simulink model "aerodinamica"  (Simulink 8.6)
settings: Solver=FixedStepAuto  StartTime=0  StopTime=150  FixedStep=1/5  RelTol=1e-3
model workspace: external: MATLAB Code (data not in the file)
values from neighbouring files (symbols this model uses):
  CD_alpha = 0.3840    (= 0.384)    [t37_data.m]
  CD_beta = [-1.5700	1.2300 ... (first row only)    [t37_data.m]
  CD_de = 0.0750    (= 0.075)    [t37_data.m]
  CD_flap = 0.0750    (= 0.075)    [t37_data.m]
  CD_ground_effect = [0.0000	0.8100 ... (first row only)    [t37_data.m]
  CD_mach = [0.0000	0.0000 ... (first row only)    [t37_data.m]
  CD_zero = [  -1.5700	1.5000 ... (first row only)    [t37_data.m]
  Cl_ail = [0.0000	0.1810 ... (first row only)    [t37_data.m]
  CL_alpha = [-0.2000	-0.6400 ... (first row only)    [t37_data.m]
  CL_alpha_dot = 2.0    (= 2)    [t37_data.m]
  Cl_beta = -0.0944    [t37_data.m]
  CL_elev = 0.5    [t37_data.m]
  CL_flap = 0.3500    (= 0.35)    [t37_data.m]
  CL_ground_effect = [0.0000	1.0610 ... (first row only)    [t37_data.m]
  Cl_p = -0.4420    (= -0.442)    [t37_data.m]
  CL_q = 4.1    [t37_data.m]
  Cl_r = 0.0926    [t37_data.m]
  Cl_rudder = 0.0150    (= 0.015)    [t37_data.m]
  Cm_alpha = -0.7000    (= -0.7)    [t37_data.m]
  Cm_alpha_dot = -6.9500    (= -6.95)    [t37_data.m]
  Cm_elev = [0.0000	-1.1200 ... (first row only)    [t37_data.m]
  Cm_q = -50.0000    (= -50)    [t37_data.m]
  Cm_zero = 0.0250    (= 0.025)    [t37_data.m]
  Cn_beta = 0.1106    [t37_data.m]
  Cn_p = -0.0243    [t37_data.m]
  Cn_r = -0.1390    (= -0.139)    [t37_data.m]
  Cn_rudder = -0.0365    [t37_data.m]
  Cnda = -0.0254    [t37_data.m]
  CY_beta = -0.3460    (= -0.346)    [t37_data.m]
  CY_p = -0.0827    [t37_data.m]
  CY_r = 0.3000    (= 0.3)    [t37_data.m]
  CY_rudder = 0.200    (= 0.2)    [t37_data.m]
  Sw = 182*0.09290304    (= 16.90835328)    [t37_data.m]
undefined symbols (not defined in the file): Bw, Cw
settings Model: Creator=willi  LastModifiedBy=willi
settings DataIOCC: SaveFormat=Dataset  SignalLoggingSaveFormat=Dataset
settings OptimizationCC: ExpressionDepthLimit=128
settings DebuggingCC: UnderspecifiedInitializationDetection=Simplified  MergeDetectMultiDrivingBlocksExec=error  SolverPrmCheckMsg=none  FcnCallInpInsideContextMsg=EnableAllAsError  StateNameClashWarn=none
settings HardwareCC: ProdBitPerPointer=64  ProdLargestAtomicFloat=Float  ProdIntDivRoundTo=Zero  ProdEndianess=LittleEndian  ProdWordSize=64  ProdHWDeviceType=Intel->x86-64 (Windows64)
settings GRTTargetCC: GeneratePreprocessorConditionals=Use local settings  CombineOutputUpdateFcns=on  GRTInterface=off

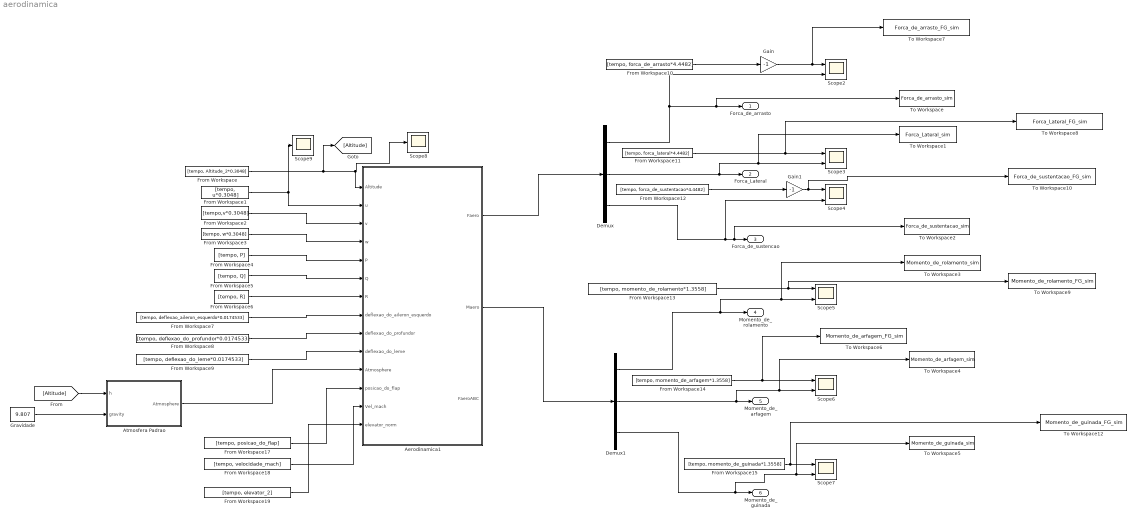
== system aerodinamica ==
  Aerodinamica1 : Subsystem  mask{flap=0, bw=Bw, cw=Cw, Sw=Sw}
      mask prompts: flap "Comando Flap (0, 1, 2 ou 3)"; bw "Comprimento da asa  - wingspan (m)"; cw "Corda media da asa (m)"; Sw "Area da asa (m2)"
  Atmosfera Padrao : Subsystem
  Demux : Demux  Outputs=3
  Demux1 : Demux  Outputs=3
  From Workspace : FromWorkspace  VariableName=[tempo, Altitude_2*0.3048]  SampleTime=0
  From Workspace1 : FromWorkspace  VariableName=[tempo, u*0.3048]  SampleTime=0
  From Workspace10 : FromWorkspace  VariableName=[tempo, forca_de_arrasto*4.4482]  SampleTime=0
  From Workspace11 : FromWorkspace  VariableName=[tempo, forca_lateral*4.4482]  SampleTime=0
  From Workspace12 : FromWorkspace  VariableName=[tempo, forca_de_sustentacao*4.4482]  SampleTime=0
  From Workspace13 : FromWorkspace  VariableName=[tempo, momento_de_rolamento*1.3558]  SampleTime=0
  From Workspace14 : FromWorkspace  VariableName=[tempo, momento_de_arfagem*1.3558]  SampleTime=0
  From Workspace15 : FromWorkspace  VariableName=[tempo, momento_de_guinada*1.3558]  SampleTime=0
  From Workspace17 : FromWorkspace  VariableName=[tempo, posicao_do_flap]  SampleTime=0
  From Workspace18 : FromWorkspace  VariableName=[tempo, velocidade_mach]  SampleTime=0
  From Workspace19 : FromWorkspace  VariableName=[tempo, elevator_2]  SampleTime=0
  From Workspace2 : FromWorkspace  VariableName=[tempo,v*0.3048]  SampleTime=0
  From Workspace3 : FromWorkspace  VariableName=[tempo, w*0.3048]  SampleTime=0
  From Workspace4 : FromWorkspace  VariableName=[tempo, P]  SampleTime=0
  From Workspace5 : FromWorkspace  VariableName=[tempo, Q]  SampleTime=0
  From Workspace6 : FromWorkspace  VariableName=[tempo, R]  SampleTime=0
  From Workspace7 : FromWorkspace  VariableName=[tempo, deflexao_aileron_esquerdo*0.0174533]  SampleTime=0
  From Workspace8 : FromWorkspace  VariableName=[tempo, deflexao_do_profundor*0.0174533]  SampleTime=0
  From Workspace9 : FromWorkspace  VariableName=[tempo, deflexao_do_leme*0.0174533]  SampleTime=0
  Gain : Gain  Gain=-1
  Gain1 : Gain  Gain=-1
  Gravidade : Constant  Value=9.807
  Scope{2..7} (6 alike) : Scope  NumInputPorts=2
  Scope8 : Scope
  Scope9 : Scope
  To Workspace : ToWorkspace  VariableName=Forca_de_arrasto_sim  SampleTime=-1
  To Workspace1 : ToWorkspace  VariableName=Forca_Lateral_sim  SampleTime=-1
  To Workspace10 : ToWorkspace  VariableName=Forca_de_sustentacao_FG_sim  SampleTime=-1
  To Workspace12 : ToWorkspace  VariableName=Momento_de_guinada_FG_sim  SampleTime=-1
  To Workspace2 : ToWorkspace  VariableName=Forca_de_sustentacao_sim  SampleTime=-1
  To Workspace3 : ToWorkspace  VariableName=Momento_de_rolamento_sim  SampleTime=-1
  To Workspace4 : ToWorkspace  VariableName=Momento_de_arfagem_sim  SampleTime=-1
  To Workspace5 : ToWorkspace  VariableName=Momento_de_guinada_sim  SampleTime=-1
  To Workspace6 : ToWorkspace  VariableName=Momento_de_arfagem_FG_sim  SampleTime=-1
  To Workspace7 : ToWorkspace  VariableName=Forca_de_arrasto_FG_sim  SampleTime=-1
  To Workspace8 : ToWorkspace  VariableName=Forca_Lateral_FG_sim  SampleTime=-1
  To Workspace9 : ToWorkspace  VariableName=Momento_de_rolamento_FG_sim  SampleTime=-1
  Forca_de_arrasto : Outport
  Forca_Lateral : Outport  Port=2
  Forca_de_sustencao : Outport  Port=3
  Momento_de_rolamento : Outport  Port=4
  Momento_de_arfagem : Outport  Port=5
  Momento_de_guinada : Outport  Port=6
  wires:
  From Workspace4/1 -> Aerodinamica1/5(P)
  From Workspace5/1 -> Aerodinamica1/6(Q)
  From Workspace6/1 -> Aerodinamica1/7(R)
  From Workspace7/1 -> Aerodinamica1/8("deflexao_do_aileron_esquerdo ")
  From Workspace8/1 -> Aerodinamica1/9("deflexao_do_profundor ")
  From Workspace9/1 -> Aerodinamica1/10(deflexao_do_leme)
  From Workspace1/1 -> Scope9/1, Aerodinamica1/2(u)
  From Workspace2/1 -> Aerodinamica1/3(v)
  From Workspace3/1 -> Aerodinamica1/4("w ")
  Gravidade/1 -> Atmosfera Padrao/2(gravity)
  Atmosfera Padrao/1(Atmosphere) -> Aerodinamica1/11(Atmosphere)
  [Altitude] -> Atmosfera Padrao/1(h)
  Aerodinamica1/1(Faero) -> Demux/1
  Demux/1 -> Scope2/2, To Workspace/1, Forca_de_arrasto/1
  Demux/2 -> To Workspace1/1, Scope3/2, Forca_Lateral/1
  Aerodinamica1/2(Maero) -> Demux1/1
  Demux/3 -> Scope4/2, To Workspace2/1, Forca_de_sustencao/1
  Demux1/2 -> Scope6/2, To Workspace4/1, Momento_de_arfagem/1
  Demux1/3 -> To Workspace5/1, Scope7/2, Momento_de_guinada/1
  Demux1/1 -> To Workspace3/1, Scope5/2, Momento_de_rolamento/1
  From Workspace14/1 -> Scope6/1, To Workspace6/1
  From Workspace15/1 -> To Workspace12/1, Scope7/1
  Gain/1 -> To Workspace7/1, Scope2/1
  From Workspace10/1 -> Gain/1
  Gain1/1 -> To Workspace10/1, Scope4/1
  From Workspace12/1 -> Gain1/1
  From Workspace11/1 -> To Workspace8/1, Scope3/1
  From Workspace17/1 -> Aerodinamica1/12(posicao_do_flap)
  From Workspace18/1 -> Aerodinamica1/13(Vel_mach)
  From Workspace13/1 -> To Workspace9/1, Scope5/1
  From Workspace/1 -> [Altitude], Scope8/1, Aerodinamica1/1(Altitude)
  From Workspace19/1 -> Aerodinamica1/14("elevator_norm ")

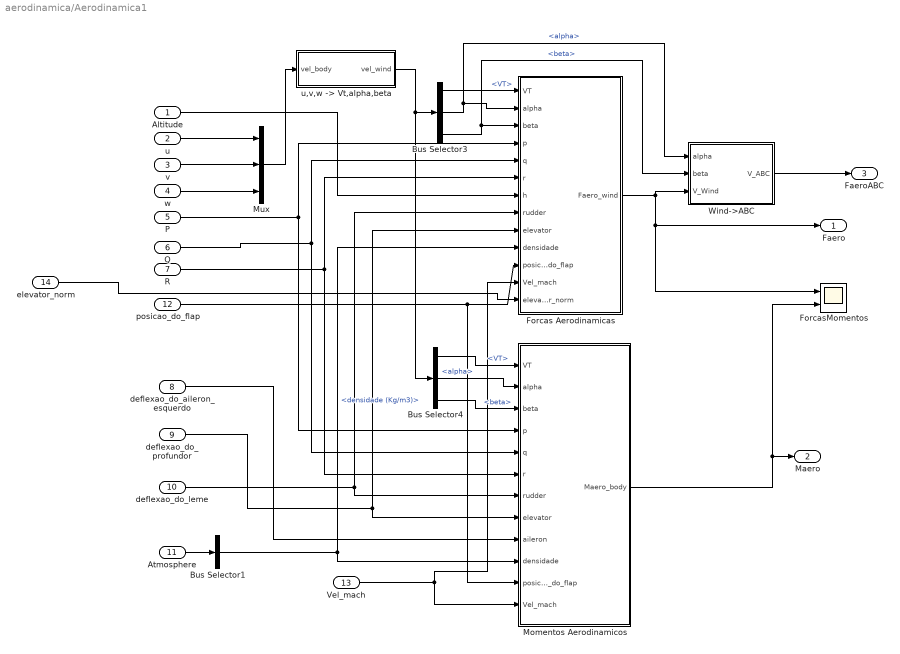
== system aerodinamica/Aerodinamica1 ==
  Altitude : Inport
  u : Inport  Port=2
  v : Inport  Port=3
  "w " : Inport  Port=4
  P : Inport  Port=5
  Q : Inport  Port=6
  R : Inport  Port=7
  "deflexao_do_aileron_esquerdo " : Inport  Port=8
  "deflexao_do_profundor " : Inport  Port=9
  deflexao_do_leme : Inport  Port=10
  Atmosphere : Inport  Port=11
  posicao_do_flap : Inport  Port=12
  Vel_mach : Inport  Port=13
  "elevator_norm " : Inport  Port=14
  Bus Selector1 : BusSelector  OutputSignals=densidade (Kg/m3)
  Bus Selector3 : BusSelector  OutputSignals=VT,alpha,beta
  Bus Selector4 : BusSelector  OutputSignals=VT,alpha,beta
  Forcas Aerodinamicas : Subsystem
  ForcasMomentos : Scope  NumInputPorts=2
  Momentos Aerodinamicos : Subsystem
  Mux : Mux  Inputs=3
  Wind->ABC : Subsystem
  "u,v,w -> Vt,alpha,beta" : Subsystem
  Faero : Outport
  Maero : Outport  Port=2
  FaeroABC : Outport  Port=3
  wires:
  Bus Selector1/1 -> Forcas Aerodinamicas/10(densidade), Momentos Aerodinamicos/10(densidade)  "<densidade (Kg/m3)>"
  Altitude/1 -> Forcas Aerodinamicas/7(h)
  P/1 -> Forcas Aerodinamicas/4(p), Momentos Aerodinamicos/4(p)
  Q/1 -> Forcas Aerodinamicas/5(q), Momentos Aerodinamicos/5(q)
  R/1 -> Forcas Aerodinamicas/6(r), Momentos Aerodinamicos/6(r)
  "deflexao_do_aileron_esquerdo "/1 -> Momentos Aerodinamicos/9(aileron)
  "deflexao_do_profundor "/1 -> Forcas Aerodinamicas/9(elevator), Momentos Aerodinamicos/8(elevator)
  deflexao_do_leme/1 -> Forcas Aerodinamicas/8(rudder), Momentos Aerodinamicos/7(rudder)
  Bus Selector3/1 -> Forcas Aerodinamicas/1(VT)  "<VT>"
  Bus Selector3/2 -> Forcas Aerodinamicas/2(alpha), Wind->ABC/1(alpha)  "<alpha>"
  Bus Selector3/3 -> Forcas Aerodinamicas/3(beta), Wind->ABC/2(beta)  "<beta>"
  Bus Selector4/1 -> Momentos Aerodinamicos/1(VT)  "<VT>"
  Bus Selector4/2 -> Momentos Aerodinamicos/2(alpha)  "<alpha>"
  Bus Selector4/3 -> Momentos Aerodinamicos/3(beta)  "<beta>"
  "u,v,w -> Vt,alpha,beta"/1(vel_wind) -> Bus Selector3/1, Bus Selector4/1
  u/1 -> Mux/1
  v/1 -> Mux/2
  "w "/1 -> Mux/3
  Mux/1 -> "u,v,w -> Vt,alpha,beta"/1(vel_body)
  Forcas Aerodinamicas/1(Faero_wind) -> Wind->ABC/3(V_Wind), ForcasMomentos/1, Faero/1
  Momentos Aerodinamicos/1(Maero_body) -> Maero/1, ForcasMomentos/2
  Atmosphere/1 -> Bus Selector1/1
  posicao_do_flap/1 -> Momentos Aerodinamicos/11(posicao_do_flap), Forcas Aerodinamicas/11("posicao_do_flap ")
  Vel_mach/1 -> Forcas Aerodinamicas/12(Vel_mach), Momentos Aerodinamicos/12(Vel_mach)
  "elevator_norm "/1 -> Forcas Aerodinamicas/13(elevator_norm)
  Wind->ABC/1(V_ABC) -> FaeroABC/1

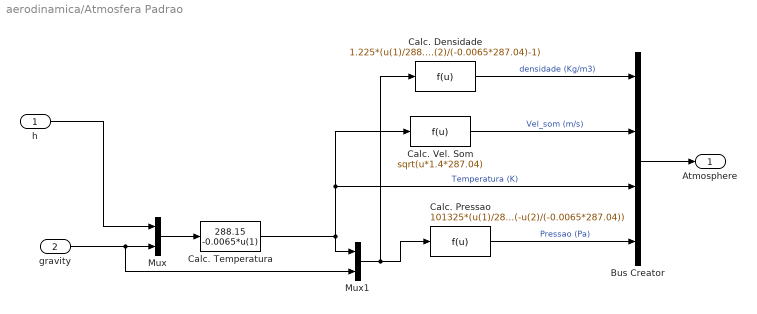
== system aerodinamica/Atmosfera Padrao ==
  h : Inport
  gravity : Inport  Port=2
  Bus Creator : BusCreator  Inputs=4
  Calc. Densidade : Fcn  Expr=1.225*(u(1)/288.15)^(-u(2)/(-0.0065*287.04)-1)
  Calc. Pressao : Fcn  Expr=101325*(u(1)/288.15)^(-u(2)/(-0.0065*287.04))
  Calc. Temperatura : Fcn  Expr=288.15 -0.0065*u(1)
  Calc. Vel. Som : Fcn  Expr=sqrt(u*1.4*287.04)
  Mux : Mux  Inputs=2
  Mux1 : Mux  Inputs=2
  Atmosphere : Outport
  wires:
  h/1 -> Mux/1
  gravity/1 -> Mux/2, Mux1/2
  Mux/1 -> Calc. Temperatura/1
  Mux1/1 -> Calc. Pressao/1, Calc. Densidade/1
  Calc. Temperatura/1 -> Mux1/1, Calc. Vel. Som/1, Bus Creator/3  "Temperatura (K)"
  Calc. Pressao/1 -> Bus Creator/4  "Pressao (Pa)"
  Calc. Densidade/1 -> Bus Creator/1  "densidade (Kg/m3)"
  Calc. Vel. Som/1 -> Bus Creator/2  "Vel_som (m/s)"
  Bus Creator/1 -> Atmosphere/1

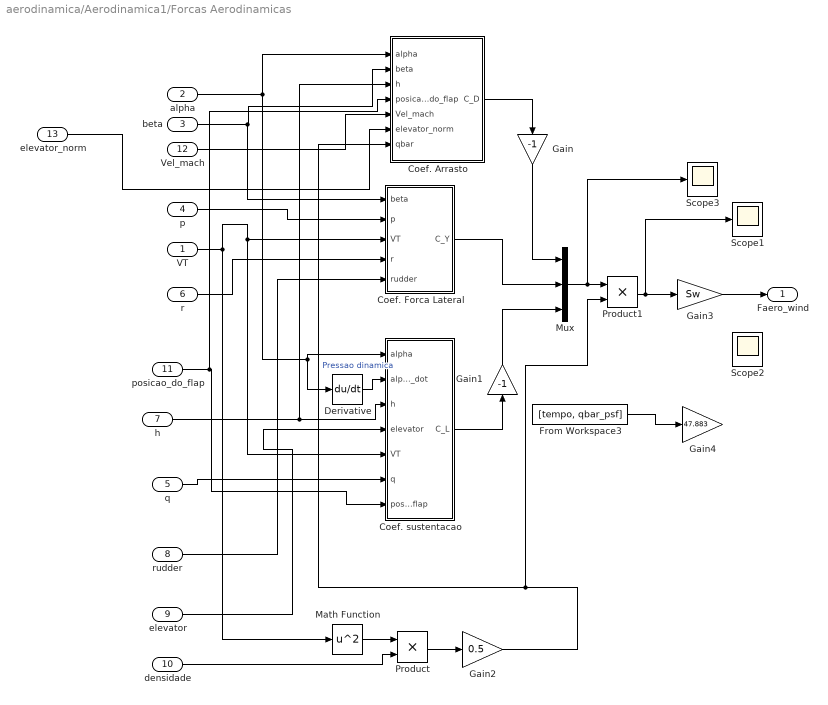
== system aerodinamica/Aerodinamica1/Forcas Aerodinamicas ==
  VT : Inport
  alpha : Inport  Port=2
  beta : Inport  Port=3
  p : Inport  Port=4
  q : Inport  Port=5
  r : Inport  Port=6
  h : Inport  Port=7
  rudder : Inport  Port=8
  elevator : Inport  Port=9
  densidade : Inport  Port=10
  "posicao_do_flap " : Inport  Port=11
  Vel_mach : Inport  Port=12
  elevator_norm : Inport  Port=13
  Coef. Arrasto : Subsystem
  Coef. Forca Lateral : Subsystem
  Coef. sustentacao : Subsystem
  Derivative : Derivative
  From Workspace3 : FromWorkspace  VariableName=[tempo, qbar_psf]  SampleTime=0
  Gain : Gain  Gain=-1  SaturateOnIntegerOverflow=on  OutDataTypeStr=Inherit: Same as input  ParamDataTypeStr=Inherit: Same as input
  Gain1 : Gain  Gain=-1  SaturateOnIntegerOverflow=on  OutDataTypeStr=Inherit: Same as input  ParamDataTypeStr=Inherit: Same as input
  Gain2 : Gain  Gain=0.5  SaturateOnIntegerOverflow=on  OutDataTypeStr=Inherit: Same as input  ParamDataTypeStr=Inherit: Same as input
  Gain3 : Gain  Gain=Sw  SaturateOnIntegerOverflow=on  OutDataTypeStr=Inherit: Same as input  ParamDataTypeStr=Inherit: Same as input
  Gain4 : Gain  Gain=47.883  SaturateOnIntegerOverflow=on  OutDataTypeStr=Inherit: Same as input  ParamDataTypeStr=Inherit: Same as input
  Math Function : Math  Operator=square  SaturateOnIntegerOverflow=on
  Mux : Mux  Inputs=3
  Product : Product  SaturateOnIntegerOverflow=on  OutDataTypeStr=Inherit: Same as first input
  Product1 : Product  SaturateOnIntegerOverflow=on  OutDataTypeStr=Inherit: Same as first input
  Scope1 : Scope
  Scope2 : Scope
  Scope3 : Scope
  Faero_wind : Outport
  wires:
  Coef. Arrasto/1(C_D) -> Gain/1
  Coef. Forca Lateral/1(C_Y) -> Mux/2
  alpha/1 -> Coef. Arrasto/1(alpha), Coef. sustentacao/1(alpha), Derivative/1
  beta/1 -> Coef. Arrasto/2(beta), Coef. Forca Lateral/1(beta)
  VT/1 -> Coef. Forca Lateral/3(VT), Coef. sustentacao/5(VT), Math Function/1
  p/1 -> Coef. Forca Lateral/2(p)
  q/1 -> Coef. sustentacao/6(q)
  r/1 -> Coef. Forca Lateral/4(r)
  h/1 -> Coef. Arrasto/3(h), Coef. sustentacao/3(h)
  rudder/1 -> Coef. Forca Lateral/5(rudder)
  elevator/1 -> Coef. sustentacao/4(elevator)
  Derivative/1 -> Coef. sustentacao/2(alpha_dot)
  Coef. sustentacao/1(C_L) -> Gain1/1
  Gain/1 -> Mux/1
  Gain1/1 -> Mux/3
  densidade/1 -> Product/2
  Math Function/1 -> Product/1
  Product/1 -> Gain2/1
  Mux/1 -> Scope3/1, Product1/1
  Product1/1 -> Scope1/1, Gain3/1
  Gain2/1 -> Product1/2, Coef. Arrasto/7(qbar)  "Pressao dinamica"
  Gain3/1 -> Faero_wind/1
  "posicao_do_flap "/1 -> Coef. Arrasto/4(posicao_do_flap), Coef. sustentacao/7("posicao_do_flap ")
  Vel_mach/1 -> Coef. Arrasto/5(Vel_mach)
  elevator_norm/1 -> Coef. Arrasto/6(elevator_norm)
  From Workspace3/1 -> Gain4/1

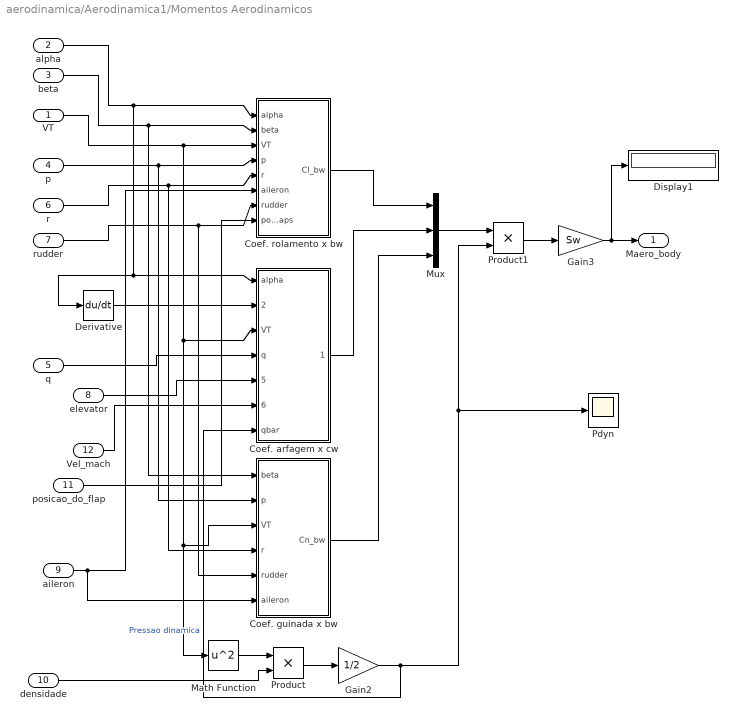
== system aerodinamica/Aerodinamica1/Momentos Aerodinamicos ==
  VT : Inport
  alpha : Inport  Port=2
  beta : Inport  Port=3
  p : Inport  Port=4
  q : Inport  Port=5
  r : Inport  Port=6
  rudder : Inport  Port=7
  elevator : Inport  Port=8
  aileron : Inport  Port=9
  densidade : Inport  Port=10
  posicao_do_flap : Inport  Port=11
  Vel_mach : Inport  Port=12
  Coef. arfagem x cw : Subsystem
  Coef. guinada x bw : Subsystem
  Coef. rolamento x bw : Subsystem
  Derivative : Derivative
  Display1 : Display
  Gain2 : Gain  Gain=1/2  SaturateOnIntegerOverflow=on  OutDataTypeStr=Inherit: Same as input  ParamDataTypeStr=Inherit: Same as input
  Gain3 : Gain  Gain=Sw  SaturateOnIntegerOverflow=on  OutDataTypeStr=Inherit: Same as input  ParamDataTypeStr=Inherit: Same as input
  Math Function : Math  Operator=square  SaturateOnIntegerOverflow=on
  Mux : Mux  Inputs=3
  Pdyn : Scope
  Product : Product  SaturateOnIntegerOverflow=on  OutDataTypeStr=Inherit: Same as first input
  Product1 : Product  SaturateOnIntegerOverflow=on  OutDataTypeStr=Inherit: Same as first input
  Maero_body : Outport
  wires:
  alpha/1 -> Coef. rolamento x bw/1(alpha), Coef. arfagem x cw/1(alpha), Derivative/1
  beta/1 -> Coef. rolamento x bw/2(beta), Coef. guinada x bw/1(beta)
  VT/1 -> Coef. rolamento x bw/3(VT), Coef. arfagem x cw/3(VT), Coef. guinada x bw/3(VT), Math Function/1
  p/1 -> Coef. rolamento x bw/4(p), Coef. guinada x bw/2(p)
  r/1 -> Coef. rolamento x bw/5(r), Coef. guinada x bw/4(r)
  Derivative/1 -> Coef. arfagem x cw/2(alpha_dot)
  q/1 -> Coef. arfagem x cw/4(q)
  rudder/1 -> Coef. rolamento x bw/7(rudder), Coef. guinada x bw/5(rudder)
  elevator/1 -> Coef. arfagem x cw/5(elevator)
  aileron/1 -> Coef. guinada x bw/6("aileron "), Coef. rolamento x bw/6(aileron)
  Mux/1 -> Product1/1
  Product1/1 -> Gain3/1
  Coef. rolamento x bw/1(Cl_bw) -> Mux/1
  Coef. arfagem x cw/1(Cm_cw) -> Mux/2
  Coef. guinada x bw/1(Cn_bw) -> Mux/3
  densidade/1 -> Product/2
  Math Function/1 -> Product/1
  Product/1 -> Gain2/1
  Gain2/1 -> Coef. arfagem x cw/7(qbar), Product1/2, Pdyn/1  "Pressao dinamica"
  Gain3/1 -> Display1/1, Maero_body/1
  posicao_do_flap/1 -> Coef. rolamento x bw/8(posicao_dos_flaps)
  Vel_mach/1 -> Coef. arfagem x cw/6(Vel_mach)

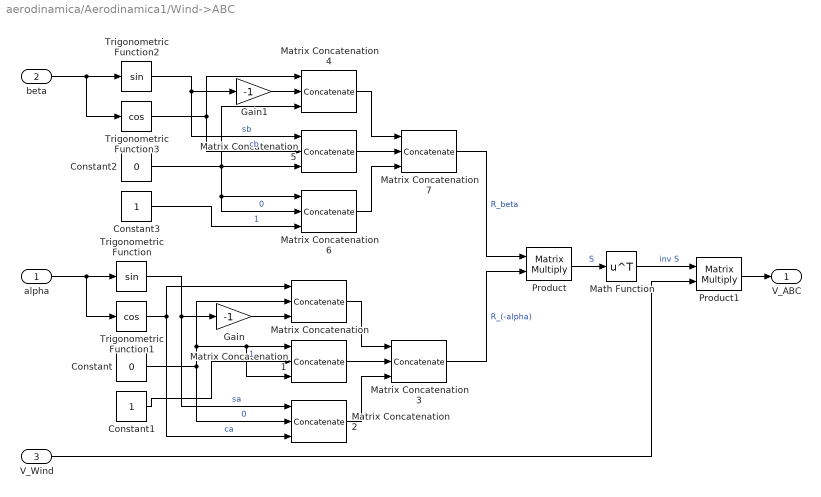
== system aerodinamica/Aerodinamica1/Wind->ABC ==
  alpha : Inport
  beta : Inport  Port=2
  V_Wind : Inport  Port=3
  Constant : Constant  Value=0
  Constant1 : Constant
  Constant2 : Constant  Value=0
  Constant3 : Constant
  Gain : Gain  Gain=-1  SaturateOnIntegerOverflow=on  OutDataTypeStr=Inherit: Same as input  ParamDataTypeStr=Inherit: Same as input
  Gain1 : Gain  Gain=-1  SaturateOnIntegerOverflow=on  OutDataTypeStr=Inherit: Same as input  ParamDataTypeStr=Inherit: Same as input
  Math Function : Math  Operator=transpose  SaturateOnIntegerOverflow=on
  Matrix Concatenation{,1..2,4..6} (6 alike) : Concatenate  NumInputs=3  Mode=Multidimensional array
  Matrix Concatenation3 : Concatenate  NumInputs=3  Mode=Multidimensional array  ConcatenateDimension=2
  Matrix Concatenation7 : Concatenate  NumInputs=3  Mode=Multidimensional array  ConcatenateDimension=2
  Product : Product  Multiplication=Matrix(*)  SaturateOnIntegerOverflow=on  OutDataTypeStr=Inherit: Same as first input
  Product1 : Product  Multiplication=Matrix(*)  SaturateOnIntegerOverflow=on  OutDataTypeStr=Inherit: Same as first input
  Trigonometric Function : Trigonometry
  Trigonometric Function1 : Trigonometry  Operator=cos
  Trigonometric Function2 : Trigonometry
  Trigonometric Function3 : Trigonometry  Operator=cos
  V_ABC : Outport
  wires:
  alpha/1 -> Trigonometric Function/1, Trigonometric Function1/1
  Trigonometric Function1/1 -> Matrix Concatenation/1, Matrix Concatenation2/3  "ca"
  Trigonometric Function/1 -> Matrix Concatenation2/1, Gain/1  "sa"
  Constant/1 -> Matrix Concatenation/2, Matrix Concatenation1/1, Matrix Concatenation1/3, Matrix Concatenation2/2  "0"
  Constant1/1 -> Matrix Concatenation1/2  "1"
  Matrix Concatenation/1 -> Matrix Concatenation3/1
  Matrix Concatenation1/1 -> Matrix Concatenation3/2
  Matrix Concatenation2/1 -> Matrix Concatenation3/3
  Product/1 -> Math Function/1  "S"
  Math Function/1 -> Product1/1  "inv S"
  Product1/1 -> V_ABC/1
  beta/1 -> Trigonometric Function2/1, Trigonometric Function3/1
  Matrix Concatenation4/1 -> Matrix Concatenation7/1
  Matrix Concatenation5/1 -> Matrix Concatenation7/2
  Matrix Concatenation6/1 -> Matrix Concatenation7/3
  Trigonometric Function3/1 -> Matrix Concatenation4/1, Matrix Concatenation5/2  "cb"
  Trigonometric Function2/1 -> Gain1/1, Matrix Concatenation5/1  "sb"
  Constant2/1 -> Matrix Concatenation4/3, Matrix Concatenation5/3, Matrix Concatenation6/1, Matrix Concatenation6/2  "0"
  Constant3/1 -> Matrix Concatenation6/3  "1"
  Matrix Concatenation7/1 -> Product/1  "R_beta"
  Matrix Concatenation3/1 -> Product/2  "R_(-alpha)"
  Gain1/1 -> Matrix Concatenation4/2
  V_Wind/1 -> Product1/2
  Gain/1 -> Matrix Concatenation/3

== system aerodinamica/Aerodinamica1/u,v,w -> Vt,alpha,beta ==
  vel_body : Inport
  Bus Creator : BusCreator  Inputs=3
  VT : Fcn  Expr=sqrt(u(1)^2+u(2)^2+u(3)^2)
  alpha : Fcn  Expr=atan2(u(3),u(1))
  beta : Fcn  Expr=atan2(u(2),sqrt(u(1)^2+u(3)^2))
  vel_wind : Outport
  wires:
  Bus Creator/1 -> vel_wind/1
  VT/1 -> Bus Creator/1  "VT"
  alpha/1 -> Bus Creator/2  "alpha"
  vel_body/1 -> alpha/1, VT/1, beta/1
  beta/1 -> Bus Creator/3  "beta"

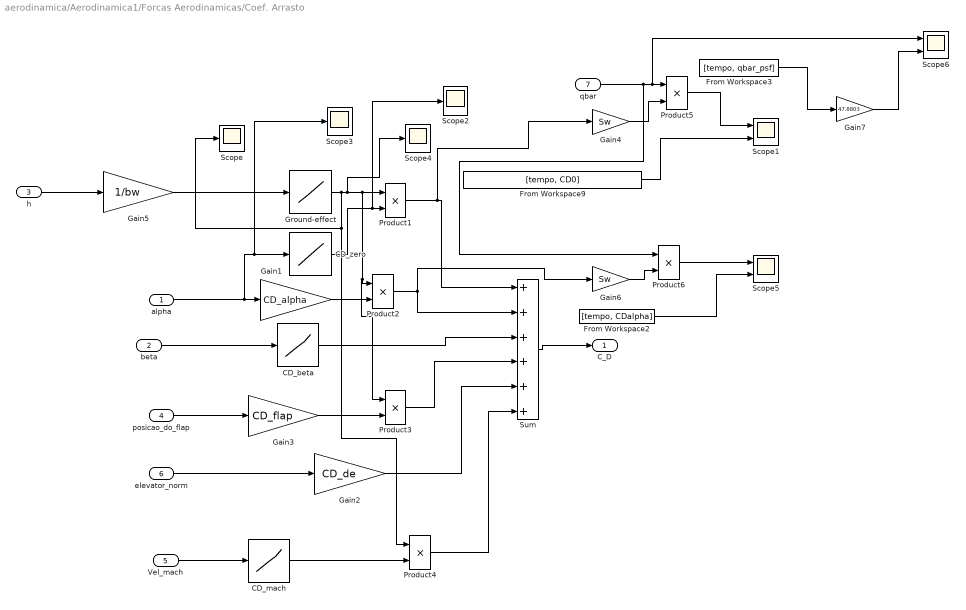
== system aerodinamica/Aerodinamica1/Forcas Aerodinamicas/Coef. Arrasto ==
  alpha : Inport
  beta : Inport  Port=2
  h : Inport  Port=3
  posicao_do_flap : Inport  Port=4
  Vel_mach : Inport  Port=5
  elevator_norm : Inport  Port=6
  qbar : Inport  Port=7
  CD_beta : Lookup  InputValues=CD_beta(:,1);  Table=CD_beta(:,2);  SaturateOnIntegerOverflow=on
  CD_mach : Lookup  InputValues=CD_mach(:,1);  Table=CD_mach(:,2);  SaturateOnIntegerOverflow=on
  CD_zero : Lookup  InputValues=CD_zero(:,1);  Table=CD_zero(:,2);  LookUpMeth=Interpolation-Use End Values  SaturateOnIntegerOverflow=on
  From Workspace2 : FromWorkspace  VariableName=[tempo, CDalpha]  SampleTime=0
  From Workspace3 : FromWorkspace  VariableName=[tempo, qbar_psf]  SampleTime=0
  From Workspace9 : FromWorkspace  VariableName=[tempo, CD0]  SampleTime=0
  Gain1 : Gain  Gain=CD_alpha  SaturateOnIntegerOverflow=on  OutDataTypeStr=Inherit: Same as input  ParamDataTypeStr=Inherit: Same as input
  Gain2 : Gain  Gain=CD_de  SaturateOnIntegerOverflow=on  OutDataTypeStr=Inherit: Same as input  ParamDataTypeStr=Inherit: Same as input
  Gain3 : Gain  Gain=CD_flap  SaturateOnIntegerOverflow=on  OutDataTypeStr=Inherit: Same as input  ParamDataTypeStr=Inherit: Same as input
  Gain4 : Gain  Gain=Sw  SaturateOnIntegerOverflow=on  OutDataTypeStr=Inherit: Same as input  ParamDataTypeStr=Inherit: Same as input
  Gain5 : Gain  Gain=1/bw  SaturateOnIntegerOverflow=on  OutDataTypeStr=Inherit: Same as input  ParamDataTypeStr=Inherit: Same as input
  Gain6 : Gain  Gain=Sw  SaturateOnIntegerOverflow=on  OutDataTypeStr=Inherit: Same as input  ParamDataTypeStr=Inherit: Same as input
  Gain7 : Gain  Gain=47.8803  SaturateOnIntegerOverflow=on  OutDataTypeStr=Inherit: Same as input  ParamDataTypeStr=Inherit: Same as input
  Ground-effect : Lookup  InputValues=CD_ground_effect(:,1);  Table=CD_ground_effect(:,2);  LookUpMeth=Interpolation-Use End Values  SaturateOnIntegerOverflow=on
  Product{1..6} (6 alike) : Product  SaturateOnIntegerOverflow=on  OutDataTypeStr=Inherit: Same as first input
  Scope{,2..4} (4 alike) : Scope
  Scope1 : Scope  NumInputPorts=2
  Scope5 : Scope  NumInputPorts=2
  Scope6 : Scope  NumInputPorts=2
  Sum : Sum  Inputs=++++++  SaturateOnIntegerOverflow=on
  C_D : Outport
  wires:
  alpha/1 -> Gain1/1, Scope3/1, CD_zero/1
  Sum/1 -> C_D/1
  CD_beta/1 -> Sum/3
  beta/1 -> CD_beta/1
  elevator_norm/1 -> Gain2/1
  posicao_do_flap/1 -> Gain3/1
  CD_zero/1 -> Scope2/1, Product1/2
  Product1/1 -> Gain4/1, Sum/1
  Gain1/1 -> Product2/2
  Product2/1 -> Sum/2, Gain6/1
  Ground-effect/1 -> Product4/1, Scope/1, Scope4/1, Product1/1, Product3/1, Product2/1
  Gain3/1 -> Product3/2
  Vel_mach/1 -> CD_mach/1
  CD_mach/1 -> Product4/2
  Product4/1 -> Sum/6
  Gain2/1 -> Sum/5
  Product3/1 -> Sum/4
  From Workspace9/1 -> Scope1/2
  Product5/1 -> Scope1/1
  Gain4/1 -> Product5/2
  Gain5/1 -> Ground-effect/1
  h/1 -> Gain5/1
  Gain6/1 -> Product6/2
  From Workspace2/1 -> Scope5/2
  Product6/1 -> Scope5/1
  qbar/1 -> Product6/1, Scope6/1, Product5/1
  From Workspace3/1 -> Gain7/1
  Gain7/1 -> Scope6/2

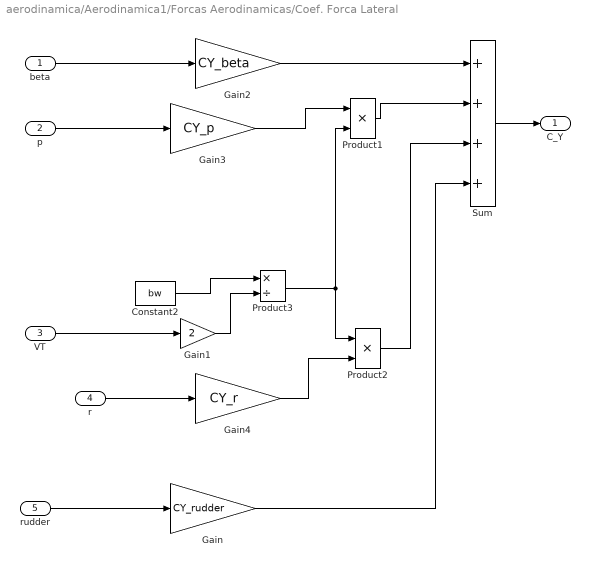
== system aerodinamica/Aerodinamica1/Forcas Aerodinamicas/Coef. Forca Lateral ==
  beta : Inport
  p : Inport  Port=2
  VT : Inport  Port=3
  r : Inport  Port=4
  rudder : Inport  Port=5
  Constant2 : Constant  Value=bw
  Gain : Gain  Gain=CY_rudder  SaturateOnIntegerOverflow=on  OutDataTypeStr=Inherit: Same as input  ParamDataTypeStr=Inherit: Same as input
  Gain1 : Gain  Gain=2  SaturateOnIntegerOverflow=on  OutDataTypeStr=Inherit: Same as input  ParamDataTypeStr=Inherit: Same as input
  Gain2 : Gain  Gain=CY_beta  SaturateOnIntegerOverflow=on  OutDataTypeStr=Inherit: Same as input  ParamDataTypeStr=Inherit: Same as input
  Gain3 : Gain  Gain=CY_p  SaturateOnIntegerOverflow=on  OutDataTypeStr=Inherit: Same as input  ParamDataTypeStr=Inherit: Same as input
  Gain4 : Gain  Gain=CY_r  SaturateOnIntegerOverflow=on  OutDataTypeStr=Inherit: Same as input  ParamDataTypeStr=Inherit: Same as input
  Product1 : Product  SaturateOnIntegerOverflow=on  OutDataTypeStr=Inherit: Same as first input
  Product2 : Product  SaturateOnIntegerOverflow=on  OutDataTypeStr=Inherit: Same as first input
  Product3 : Product  Inputs=*/  SaturateOnIntegerOverflow=on  OutDataTypeStr=Inherit: Same as first input
  Sum : Sum  Inputs=++++  SaturateOnIntegerOverflow=on
  C_Y : Outport
  wires:
  beta/1 -> Gain2/1
  Sum/1 -> C_Y/1
  Gain2/1 -> Sum/1
  Product1/1 -> Sum/2
  Gain3/1 -> Product1/1
  VT/1 -> Gain1/1
  Gain1/1 -> Product3/2
  Constant2/1 -> Product3/1
  Product3/1 -> Product1/2, Product2/1
  Product2/1 -> Sum/3
  r/1 -> Gain4/1
  Gain/1 -> Sum/4
  rudder/1 -> Gain/1
  Gain4/1 -> Product2/2
  p/1 -> Gain3/1

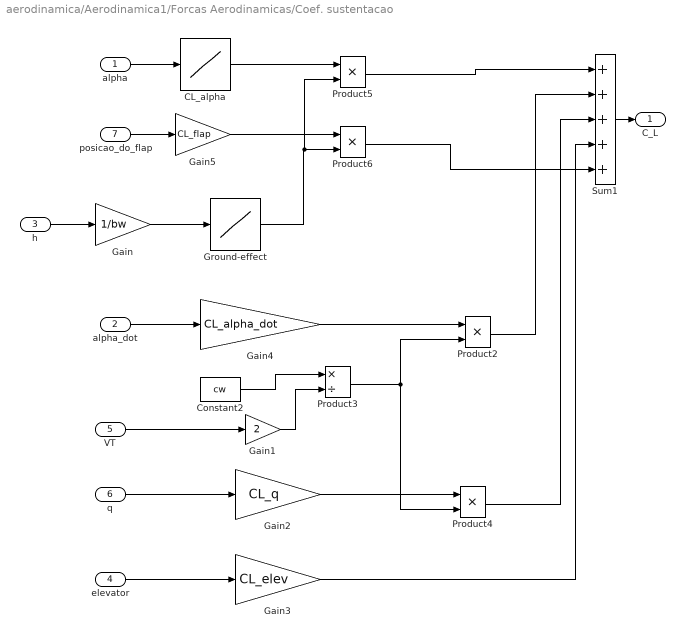
== system aerodinamica/Aerodinamica1/Forcas Aerodinamicas/Coef. sustentacao ==
  alpha : Inport
  alpha_dot : Inport  Port=2
  h : Inport  Port=3
  elevator : Inport  Port=4
  VT : Inport  Port=5
  q : Inport  Port=6
  "posicao_do_flap " : Inport  Port=7
  CL_alpha : Lookup  InputValues=CL_alpha(:,1);  Table=CL_alpha(:,2);  LookUpMeth=Interpolation-Use End Values  SaturateOnIntegerOverflow=on
  Constant2 : Constant  Value=cw
  Gain : Gain  Gain=1/bw  SaturateOnIntegerOverflow=on  OutDataTypeStr=Inherit: Same as input  ParamDataTypeStr=Inherit: Same as input
  Gain1 : Gain  Gain=2  SaturateOnIntegerOverflow=on  OutDataTypeStr=Inherit: Same as input  ParamDataTypeStr=Inherit: Same as input
  Gain2 : Gain  Gain=CL_q  SaturateOnIntegerOverflow=on  OutDataTypeStr=Inherit: Same as input  ParamDataTypeStr=Inherit: Same as input
  Gain3 : Gain  Gain=CL_elev  SaturateOnIntegerOverflow=on  OutDataTypeStr=Inherit: Same as input  ParamDataTypeStr=Inherit: Same as input
  Gain4 : Gain  Gain=CL_alpha_dot  SaturateOnIntegerOverflow=on  OutDataTypeStr=Inherit: Same as input  ParamDataTypeStr=Inherit: Same as input
  Gain5 : Gain  Gain=CL_flap  SaturateOnIntegerOverflow=on  OutDataTypeStr=Inherit: Same as input  ParamDataTypeStr=Inherit: Same as input
  Ground-effect : Lookup  InputValues=CL_ground_effect(:,1);  Table=CL_ground_effect(:,2);  LookUpMeth=Interpolation-Use End Values  SaturateOnIntegerOverflow=on
  Product{2,4..6} (4 alike) : Product  SaturateOnIntegerOverflow=on  OutDataTypeStr=Inherit: Same as first input
  Product3 : Product  Inputs=*/  SaturateOnIntegerOverflow=on  OutDataTypeStr=Inherit: Same as first input
  Sum1 : Sum  Inputs=+++++  SaturateOnIntegerOverflow=on
  C_L : Outport
  wires:
  alpha/1 -> CL_alpha/1
  Gain/1 -> Ground-effect/1
  h/1 -> Gain/1
  Sum1/1 -> C_L/1
  Gain4/1 -> Product2/1
  VT/1 -> Gain1/1
  Gain1/1 -> Product3/2
  Constant2/1 -> Product3/1
  Product2/1 -> Sum1/2
  Product3/1 -> Product2/2, Product4/2
  Gain2/1 -> Product4/1
  Product4/1 -> Sum1/3
  q/1 -> Gain2/1
  elevator/1 -> Gain3/1
  Gain3/1 -> Sum1/4
  alpha_dot/1 -> Gain4/1
  CL_alpha/1 -> Product5/1
  Ground-effect/1 -> Product5/2, Product6/2
  "posicao_do_flap "/1 -> Gain5/1
  Gain5/1 -> Product6/1
  Product5/1 -> Sum1/1
  Product6/1 -> Sum1/5

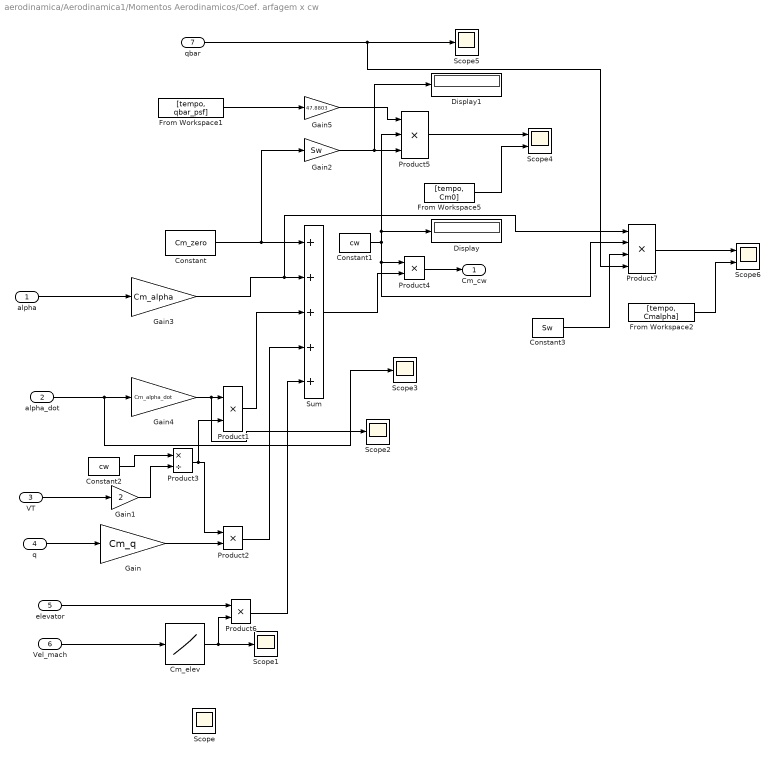
== system aerodinamica/Aerodinamica1/Momentos Aerodinamicos/Coef. arfagem x cw ==
  alpha : Inport
  alpha_dot : Inport  Port=2
  VT : Inport  Port=3
  q : Inport  Port=4
  elevator : Inport  Port=5
  Vel_mach : Inport  Port=6
  qbar : Inport  Port=7
  Cm_elev : Lookup  InputValues=Cm_elev(:,1);  Table=Cm_elev(:,2);  SaturateOnIntegerOverflow=on
  Constant : Constant  Value=Cm_zero
  Constant1 : Constant  Value=cw
  Constant2 : Constant  Value=cw
  Constant3 : Constant  Value=Sw
  Display : Display
  Display1 : Display
  From Workspace1 : FromWorkspace  VariableName=[tempo, qbar_psf]  SampleTime=0
  From Workspace2 : FromWorkspace  VariableName=[tempo, Cmalpha]  SampleTime=0
  From Workspace5 : FromWorkspace  VariableName=[tempo, Cm0]  SampleTime=0
  Gain : Gain  Gain=Cm_q  SaturateOnIntegerOverflow=on  OutDataTypeStr=Inherit: Same as input  ParamDataTypeStr=Inherit: Same as input
  Gain1 : Gain  Gain=2  SaturateOnIntegerOverflow=on  OutDataTypeStr=Inherit: Same as input  ParamDataTypeStr=Inherit: Same as input
  Gain2 : Gain  Gain=Sw  SaturateOnIntegerOverflow=on  OutDataTypeStr=Inherit: Same as input  ParamDataTypeStr=Inherit: Same as input
  Gain3 : Gain  Gain=Cm_alpha  SaturateOnIntegerOverflow=on  OutDataTypeStr=Inherit: Same as input  ParamDataTypeStr=Inherit: Same as input
  Gain4 : Gain  Gain=Cm_alpha_dot  SaturateOnIntegerOverflow=on  OutDataTypeStr=Inherit: Same as input  ParamDataTypeStr=Inherit: Same as input
  Gain5 : Gain  Gain=47.8803  SaturateOnIntegerOverflow=on  OutDataTypeStr=Inherit: Same as input  ParamDataTypeStr=Inherit: Same as input
  Product{1..2,4,6} (4 alike) : Product  Inputs=**  SaturateOnIntegerOverflow=on  OutDataTypeStr=Inherit: Same as first input
  Product3 : Product  Inputs=*/  SaturateOnIntegerOverflow=on  OutDataTypeStr=Inherit: Same as first input
  Product5 : Product  Inputs=***  SaturateOnIntegerOverflow=on  OutDataTypeStr=Inherit: Same as first input
  Product7 : Product  Inputs=****  SaturateOnIntegerOverflow=on  OutDataTypeStr=Inherit: Same as first input
  Scope{,1..3,5} (5 alike) : Scope
  Scope4 : Scope  NumInputPorts=2
  Scope6 : Scope  NumInputPorts=2
  Sum : Sum  Inputs=+++++  SaturateOnIntegerOverflow=on
  Cm_cw : Outport
  wires:
  alpha/1 -> Gain3/1
  Constant1/1 -> Display/1, Product5/2, Product7/2, Product4/1
  Sum/1 -> Product4/2
  Product4/1 -> Cm_cw/1
  VT/1 -> Gain1/1
  Gain1/1 -> Product3/2
  Constant2/1 -> Product3/1
  q/1 -> Gain/1
  Gain/1 -> Product2/2
  Product2/1 -> Sum/4
  Gain3/1 -> Product7/1, Sum/2
  Gain4/1 -> Scope2/1, Product1/1
  alpha_dot/1 -> Scope3/1, Gain4/1
  Product3/1 -> Product2/1, Product1/2
  elevator/1 -> Product6/1
  Cm_elev/1 -> Scope1/1, Product6/2
  Constant/1 -> Gain2/1, Sum/1
  Product1/1 -> Sum/3
  Product6/1 -> Sum/5
  Vel_mach/1 -> Cm_elev/1
  Gain2/1 -> Display1/1, Product5/3
  Product5/1 -> Scope4/1
  From Workspace5/1 -> Scope4/2
  qbar/1 -> Product7/4, Scope5/1
  From Workspace1/1 -> Gain5/1
  Gain5/1 -> Product5/1
  Constant3/1 -> Product7/3
  Product7/1 -> Scope6/1
  From Workspace2/1 -> Scope6/2

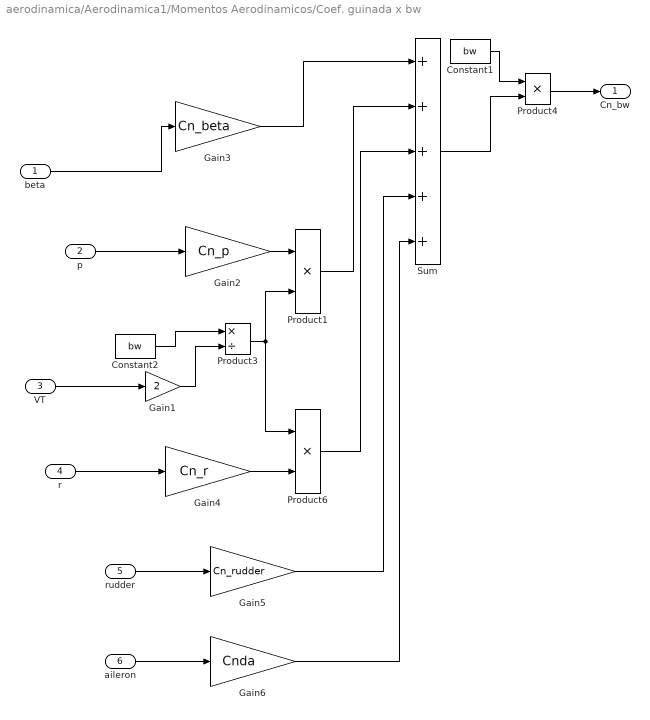
== system aerodinamica/Aerodinamica1/Momentos Aerodinamicos/Coef. guinada x bw ==
  beta : Inport
  p : Inport  Port=2
  VT : Inport  Port=3
  r : Inport  Port=4
  rudder : Inport  Port=5
  "aileron " : Inport  Port=6
  Constant1 : Constant  Value=bw
  Constant2 : Constant  Value=bw
  Gain1 : Gain  Gain=2  SaturateOnIntegerOverflow=on  OutDataTypeStr=Inherit: Same as input  ParamDataTypeStr=Inherit: Same as input
  Gain2 : Gain  Gain=Cn_p  SaturateOnIntegerOverflow=on  OutDataTypeStr=Inherit: Same as input  ParamDataTypeStr=Inherit: Same as input
  Gain3 : Gain  Gain=Cn_beta  SaturateOnIntegerOverflow=on  OutDataTypeStr=Inherit: Same as input  ParamDataTypeStr=Inherit: Same as input
  Gain4 : Gain  Gain=Cn_r  SaturateOnIntegerOverflow=on  OutDataTypeStr=Inherit: Same as input  ParamDataTypeStr=Inherit: Same as input
  Gain5 : Gain  Gain=Cn_rudder  SaturateOnIntegerOverflow=on  OutDataTypeStr=Inherit: Same as input  ParamDataTypeStr=Inherit: Same as input
  Gain6 : Gain  Gain=Cnda  SaturateOnIntegerOverflow=on  OutDataTypeStr=Inherit: Same as input  ParamDataTypeStr=Inherit: Same as input
  Product1 : Product  Inputs=**  SaturateOnIntegerOverflow=on  OutDataTypeStr=Inherit: Same as first input
  Product3 : Product  Inputs=*/  SaturateOnIntegerOverflow=on  OutDataTypeStr=Inherit: Same as first input
  Product4 : Product  Inputs=**  SaturateOnIntegerOverflow=on  OutDataTypeStr=Inherit: Same as first input
  Product6 : Product  Inputs=**  SaturateOnIntegerOverflow=on  OutDataTypeStr=Inherit: Same as first input
  Sum : Sum  Inputs=+++++  SaturateOnIntegerOverflow=on
  Cn_bw : Outport
  wires:
  Constant1/1 -> Product4/1
  Sum/1 -> Product4/2
  Product4/1 -> Cn_bw/1
  VT/1 -> Gain1/1
  Gain1/1 -> Product3/2
  Constant2/1 -> Product3/1
  beta/1 -> Gain3/1
  Gain3/1 -> Sum/1
  Product3/1 -> Product1/2, Product6/1
  Product1/1 -> Sum/2
  r/1 -> Gain4/1
  Product6/1 -> Sum/3
  rudder/1 -> Gain5/1
  Gain2/1 -> Product1/1
  Gain4/1 -> Product6/2
  Gain5/1 -> Sum/4
  p/1 -> Gain2/1
  "aileron "/1 -> Gain6/1
  Gain6/1 -> Sum/5

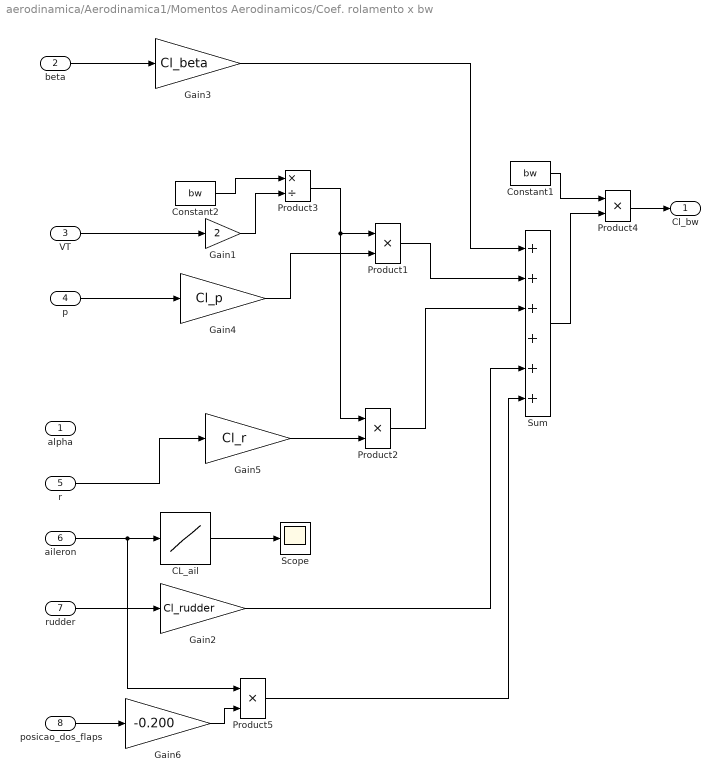
== system aerodinamica/Aerodinamica1/Momentos Aerodinamicos/Coef. rolamento x bw ==
  alpha : Inport
  beta : Inport  Port=2
  VT : Inport  Port=3
  p : Inport  Port=4
  r : Inport  Port=5
  aileron : Inport  Port=6
  rudder : Inport  Port=7
  posicao_dos_flaps : Inport  Port=8
  CL_ail : Lookup  InputValues=Cl_ail(:,1);  Table=Cl_ail(:,2);  SaturateOnIntegerOverflow=on
  Constant1 : Constant  Value=bw
  Constant2 : Constant  Value=bw
  Gain1 : Gain  Gain=2  SaturateOnIntegerOverflow=on  OutDataTypeStr=Inherit: Same as input  ParamDataTypeStr=Inherit: Same as input
  Gain2 : Gain  Gain=Cl_rudder  SaturateOnIntegerOverflow=on  OutDataTypeStr=Inherit: Same as input  ParamDataTypeStr=Inherit: Same as input
  Gain3 : Gain  Gain=Cl_beta  SaturateOnIntegerOverflow=on  OutDataTypeStr=Inherit: Same as input  ParamDataTypeStr=Inherit: Same as input
  Gain4 : Gain  Gain=Cl_p  SaturateOnIntegerOverflow=on  OutDataTypeStr=Inherit: Same as input  ParamDataTypeStr=Inherit: Same as input
  Gain5 : Gain  Gain=Cl_r  SaturateOnIntegerOverflow=on  OutDataTypeStr=Inherit: Same as input  ParamDataTypeStr=Inherit: Same as input
  Gain6 : Gain  Gain=-0.200  SaturateOnIntegerOverflow=on  OutDataTypeStr=Inherit: Same as input  ParamDataTypeStr=Inherit: Same as input
  Product1 : Product  SaturateOnIntegerOverflow=on  OutDataTypeStr=Inherit: Same as first input
  Product2 : Product  SaturateOnIntegerOverflow=on  OutDataTypeStr=Inherit: Same as first input
  Product3 : Product  Inputs=*/  SaturateOnIntegerOverflow=on  OutDataTypeStr=Inherit: Same as first input
  Product4 : Product  Inputs=**  SaturateOnIntegerOverflow=on  OutDataTypeStr=Inherit: Same as first input
  Product5 : Product  SaturateOnIntegerOverflow=on  OutDataTypeStr=Inherit: Same as first input
  Scope : Scope
  Sum : Sum  Inputs=++++++  SaturateOnIntegerOverflow=on
  Cl_bw : Outport
  wires:
  VT/1 -> Gain1/1
  Gain1/1 -> Product3/2
  Constant2/1 -> Product3/1
  Product3/1 -> Product1/1, Product2/1
  Gain4/1 -> Product1/2
  r/1 -> Gain5/1
  aileron/1 -> Product5/1, CL_ail/1
  rudder/1 -> Gain2/1
  Product1/1 -> Sum/2
  Product2/1 -> Sum/3
  Gain2/1 -> Sum/5
  Constant1/1 -> Product4/1
  Sum/1 -> Product4/2
  Product4/1 -> Cl_bw/1
  Gain5/1 -> Product2/2
  beta/1 -> Gain3/1
  Gain3/1 -> Sum/1
  p/1 -> Gain4/1
  Gain6/1 -> Product5/2
  posicao_dos_flaps/1 -> Gain6/1
  Product5/1 -> Sum/6
  CL_ail/1 -> Scope/1
